simulink model "Optimized_Quadrotor_Trajectory_PID_Control"  (R2021b)
settings: Solver=ode3  StartTime=0.0  StopTime=70  FixedStep=1e-3  RelTol=1e-3
libraries: vrlib x2
(part 2 of 2)

== matlab function Optimized_Quadrotor_Trajectory_PID_Control/Subsystem1/MATLAB Function1 ==
  data: Fz input; Tau input; V input; Omega input; eta input; dV output; dOmega output
function [dV,dOmega] = fcn(Fz,Tau,V,Omega,eta)

Parametros = [  % Manufacturer
   1.79
   0.03
   0.00
   0.00
   0.03
   0.00
   0.04];

% Parametros = [  % 14-Jun-2019_18-33-20 T1E1
%    1.829678147298636
%    0.010093518395732
%   -0.000587374456966
%    0.003051684795895
%    0.020934240830821
%    0.000179364005119
%    0.105471993294800];

% Parametros = [  % 14-Jun-2019_18-36-38 T1E2
%    1.818755164320559
%    0.015372527142417
%   -0.003406485346485
%    0.002083178012305
%    0.019512061907602
%   -0.000620131329515
%    0.111022013170028];

% Parametros = [  % 20-Jun-2019_09-03-15 T2E1
%    1.814045169635898
%    0.009638937954855
%    0.000236321278316
%   -0.000440168241711
%    0.016271439845061
%   -0.001384767379204
%    0.084705097036282];

% Parametros = [  % 20-Jun-2019_09-07-19 T2E2
%    1.816449038428290
%    0.013453840218778
%    0.002848965863275
%   -0.000914261709212
%    0.013755836350366
%   -0.000964489425951
%    0.091879162538837];

% Parametros = [  % 20-Jun-2019_09-28-11 T2E3
%    1.808642457560659
%    0.011646527138149
%    0.002508639181441
%   -0.000559939657039
%    0.022996229568014
%   -0.000675956378368
%    0.091082362761357];

% Parametros = [  % 03-Jul-2019_11-44-51 T3E1
%    1.778776027879048
%    0.015880402609160
%    0.000921132391568
%    0.002043873620352
%    0.010672144758772
%    0.002653429938916
%    0.091385789990198];

% Parametros = [  % 03-Jul-2019_11-48-21 T3E2
%    1.785869074384763
%    0.010552973622277
%   -0.000116219938120
%    0.001165427701030
%    0.015552279444504
%    0.003206150645022
%    0.098577562109087];

% Parametros = [  % 03-Jul-2019_11-57-23 T4E1
%    1.737611579857987
%    0.022499330829682
%   -0.000701639931302
%   -0.000274522399987
%    0.019053102352100
%    0.002501032319942
%    0.095393148394978];

% Parametros = [  % 03-Jul-2019_12-05-29 T4E2
%    1.753732724782751
%    0.019833420574395
%   -0.001838988010042
%    0.000664719548222
%    0.017802221622542
%    0.002855090149509
%    0.104254468680096];

 m = Parametros(1); %Masa del quadrotor [Kg]
 g = 9.81;  %Accel. Gravitacional [m/s^2]
 Tensor = Parametros(2:7);
ez = [0;0;1];


 I = [Tensor(1)  Tensor(2)  Tensor(3);
      Tensor(2)  Tensor(4)  Tensor(5);
      Tensor(3)  Tensor(5)  Tensor(6)];

phi = eta(1);
tta = eta(2);
psi = eta(3);

R = [cos(psi)*cos(tta)  cos(psi)*sin(tta)*sin(phi)-sin(psi)*cos(phi)  cos(psi)*cos(phi)*sin(tta)+sin(psi)*sin(phi)
     sin(psi)*cos(tta)  sin(phi)*sin(tta)*sin(psi)+cos(psi)*cos(phi)  sin(tta)*sin(psi)*cos(phi)-cos(psi)*sin(phi)
     -sin(tta)          cos(tta)*sin(phi)                            cos(tta)*cos(phi)];

SOmega = [0        -Omega(3)  Omega(2);
          Omega(3)  0        -Omega(1);
         -Omega(2)  Omega(1)  0];
     
G = m*g*R'*ez;

dV     = (Fz*ez - m*SOmega*V - G)/m;
dOmega = I\(Tau - SOmega*I*Omega);

== matlab function Optimized_Quadrotor_Trajectory_PID_Control/PID Controller/Position Controller ==
  data: ep input; iep input; Fz output; dep input; ddpd input; eta input; phid output; ttad output; psid input
function [Fz,phid,ttad] = fcn(ep, iep, dep, ddpd, eta, psid)

  m = 1.79; %Masa del quadrotor [Kg]
  g = 9.81;  %Accel. Gravitacional [m/s^2]

kpx = 11.5;
kpy = 10.0;
kpz = 10.5;

kdx = 5.5;
kdy = 5.0;
kdz = 6.0;

kix = 0.04;
kiy = 0.04;
kiz = 1.3;

phi = eta(1);
tta = eta(2);

ex = ep(1);
ey = ep(2);
ez = ep(3);

iex = iep(1);
iey = iep(2);
iez = iep(3);

dex = dep(1);
dey = dep(2);
dez = dep(3);

ddxd = ddpd(1);
ddyd = ddpd(2);
ddzd = ddpd(3);

fpz = m*ddzd + m*g + kpz*ez + kdz*dez + kiz*iez;
Fz = fpz/(cos(phi)*cos(tta));

fpx = m*ddxd + kpx*ex + kdx*dex + kix*iex;
fpy = m*ddyd + kpy*ey + kdy*dey + kiy*iey;

ttad = atan((fpy*sin(psid) + fpx*cos(psid))/fpz);
phid = atan(cos(ttad)*(fpx*sin(psid) - fpy*cos(psid))/fpz);
